simulink model "CF012A_GmStrtStop"  (R2013b)
settings: Solver=FixedStepDiscrete  SolverMode=SingleTasking  StartTime=0.0  StopTime=1  FixedStep=0.002  RelTol=1e-3
values from neighbouring files (symbols this model uses):
  CNV100MICROSECTOMILLISEC_MILLISECPERCNT_F32 = DataDict.Constant    [CF012A_GmStrtStop_DataDict.m]
  DISMOD_CNT_U08 = DataDict.Constant    [CF012A_GmStrtStop_DataDict.m]
  DISMODRATE_ULSPERSEC_F32 = DataDict.Constant    [CF012A_GmStrtStop_DataDict.m]
  FLTMOD_CNT_U08 = DataDict.Constant    [CF012A_GmStrtStop_DataDict.m]
  GmStrtStopEna = DataDict.Calibration    [CF012A_GmStrtStop_DataDict.m]
  GmStrtStopFltRateLim = DataDict.Calibration    [CF012A_GmStrtStop_DataDict.m]
  GmStrtStopMod1ToStopRateLim = DataDict.Calibration    [CF012A_GmStrtStop_DataDict.m]
  GmStrtStopNormRateLim = DataDict.Calibration    [CF012A_GmStrtStop_DataDict.m]
  GmStrtStopNormToMod1RateLim = DataDict.Calibration    [CF012A_GmStrtStop_DataDict.m]
  GmStrtStopStopAndMod2RateLim = DataDict.Calibration    [CF012A_GmStrtStop_DataDict.m]
  GmStrtStopStopMod1Tmr = DataDict.Calibration    [CF012A_GmStrtStop_DataDict.m]
  GmStrtStopStopMod2Tmr = DataDict.Calibration    [CF012A_GmStrtStop_DataDict.m]
  MOD1_CNT_U08 = DataDict.Constant    [CF012A_GmStrtStop_DataDict.m]
  MOD2_CNT_U08 = DataDict.Constant    [CF012A_GmStrtStop_DataDict.m]
  NORMMOD_CNT_U08 = DataDict.Constant    [CF012A_GmStrtStop_DataDict.m]
  STOPMOD_CNT_U08 = DataDict.Constant    [CF012A_GmStrtStop_DataDict.m]
  STRTSTOPRATEHILIM_ULSPERSEC_F32 = DataDict.Constant    [CF012A_GmStrtStop_DataDict.m]
  STRTSTOPRATELOWRLIM_ULSPERSEC_F32 = DataDict.Constant    [CF012A_GmStrtStop_DataDict.m]
  STRTSTOPSCAHILIM_ULS_F32 = DataDict.Constant    [CF012A_GmStrtStop_DataDict.m]
  STRTSTOPSCALOWRLIM_ULS_F32 = DataDict.Constant    [CF012A_GmStrtStop_DataDict.m]
undefined symbols (not defined in the file or in its folder): u2, u3, u4, u5
libraries: FixdToFloat x2, NxtrLim x2, simulink x2
(part 3 of 4)

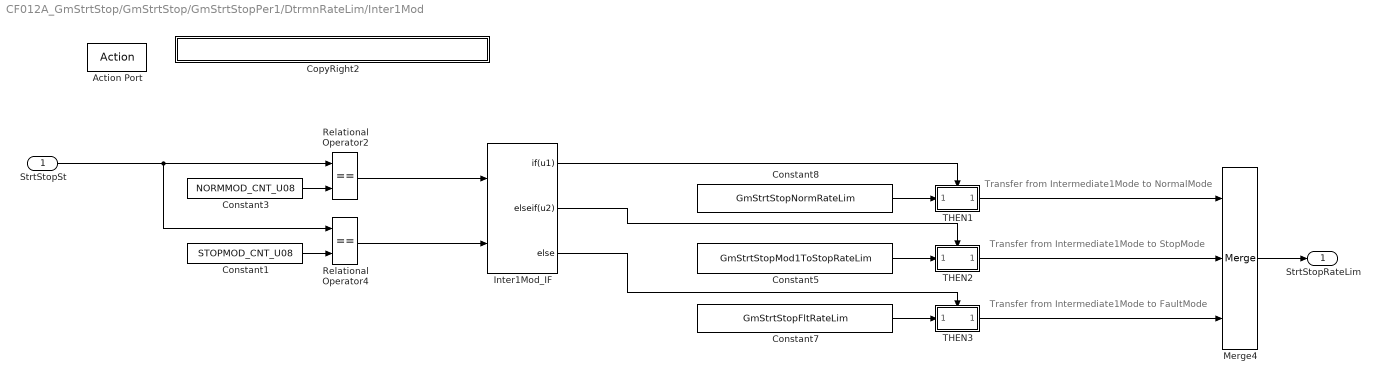
== system CF012A_GmStrtStop/GmStrtStop/GmStrtStopPer1/DtrmnRateLim/Inter1Mod ==
  note: Transfer from Intermediate1Mode to NormalMode
  note: Transfer from Intermediate1Mode to StopMode
  note: Transfer from Intermediate1Mode to FaultMode
  StrtStopSt : Inport  RequirementInfo="{'linktype_rmi_doors' '0000c6e0 (/GM T1XX/SubSystem Specifications/Customer Functions/CF012 12V Start Stop)' '#148' 'true' 'REQ:  148' '' } %GIDa_f5330e2e_2d56_43f6_8853_8fc29ce50161"
  Action Port : ActionPort  ActionType=elseif
  Constant1 : Constant  RequirementInfo="{'linktype_rmi_doors' '0000c6e0 (/GM T1XX/SubSystem Specifications/Customer Functions/CF012 12V Start Stop)' '#188' 'true' 'REQ:  188' '' } %GIDa_86f023b6_4738_45d0_828d_c113ed7026e9"  Value=STOPMOD_CNT_U08
  Constant3 : Constant  RequirementInfo="{'linktype_rmi_doors' '0000c6e0 (/GM T1XX/SubSystem Specifications/Customer Functions/CF012 12V Start Stop)' '#148' 'true' 'REQ:  148' '' } %GIDa_17212798_c997_48f1_a715_ee95a1adc504"  Value=NORMMOD_CNT_U08
  Constant5 : Constant  RequirementInfo="{'linktype_rmi_doors' '0000c6e0 (/GM T1XX/SubSystem Specifications/Customer Functions/CF012 12V Start Stop)' '#188' 'true' 'REQ:  188' '' } %GIDa_c9c10e63_8319_420b_bd57_9b2abca2294d"  Value=GmStrtStopMod1ToStopRateLim  OutDataTypeStr=single
  Constant7 : Constant  RequirementInfo="{'linktype_rmi_doors' '0000c6e0 (/GM T1XX/SubSystem Specifications/Customer Functions/CF012 12V Start Stop)' '#196' 'true' 'REQ:  196' '' } %GIDa_3c95a9bc_424d_44d0_af3d_886c4295a172"  Value=GmStrtStopFltRateLim  OutDataTypeStr=single
  Constant8 : Constant  RequirementInfo="{'linktype_rmi_doors' '0000c6e0 (/GM T1XX/SubSystem Specifications/Customer Functions/CF012 12V Start Stop)' '#148' 'true' 'REQ:  148' '' } %GIDa_b1015bd6_7f60_4122_9076_9e894186dcc2"  Value=GmStrtStopNormRateLim  OutDataTypeStr=single
  CopyRight2 : Subsystem  Description=|  mask(Copyright Information){none=on}
      | Copyright info block.                                               
      |                                                                     
      | Place copyright information at the top of every subsystem in design.
      mask prompts: none "No parameters"
      mask help: Place copyright information at the top of every subsystem in design.
      mask Display:
      | NxtrConf = 'Nexteer Confidential';
      | 
      | sys = bdroot; %handle for the current model ("system")
      | first = get_param(sys,'Created');
      | if(isempty(first))
      |     first = datestr(now,'yyyy');
      | else
      |     first = first(end-3:end);  %year is last four digits
      | end
      | 
      | last = get_param(sys,'LastModifiedDate');
      | if isempty(last)
      |     last = datestr(now,'yyyy');
      | else
      |     last = last(end-3:end);
      | end
      | 
      | if strcmp(first,last)
      |     fprintf('%s -- Copyright %s Nexteer',NxtrConf,first)
      | else
      |     fprintf('%s -- %s%s- %s Nexteer',NxtrConf,char(169),first,last)
      | end
  Inter1Mod_IF : If  RequirementInfo="{'linktype_rmi_doors' '0000c6e0 (/GM T1XX/SubSystem Specifications/Customer Functions/CF012 12V Start Stop)' '#148' 'true' 'REQ:  148' '' ; 'linktype_rmi_doors' '0000c6e0 (/GM T1XX/SubSystem Specifications/Customer Functions/CF012 12V Start Stop)' '#188' 'true' 'REQ:  188' '' ; 'linktype_rmi_doors' '0000c6e0 (/GM T1XX/SubSystem Specifications/Customer Functions/CF012 12V Start Stop)' '#196' 'true' 'REQ:  196' '' } %GIDa_bee18bf5_7cb1_484e_b310_4188a01c4900"  NumInputs=2  IfExpression=u1  ElseIfExpressions=u2
  Merge4 : Merge  RequirementInfo="{'linktype_rmi_doors' '0000c6e0 (/GM T1XX/SubSystem Specifications/Customer Functions/CF012 12V Start Stop)' '#148' 'true' 'REQ:  148' '' } %GIDa_b0435a17_739c_4c31_ac1a_85f448c6e576"  Inputs=3
  Relational Operator2 : RelationalOperator  RequirementInfo="{'linktype_rmi_doors' '0000c6e0 (/GM T1XX/SubSystem Specifications/Customer Functions/CF012 12V Start Stop)' '#148' 'true' 'REQ:  148' '' } %GIDa_db00afd9_8b52_48d0_ab8e_5bbb76a40030"  Operator===  OutDataTypeStr=boolean
  Relational Operator4 : RelationalOperator  RequirementInfo="{'linktype_rmi_doors' '0000c6e0 (/GM T1XX/SubSystem Specifications/Customer Functions/CF012 12V Start Stop)' '#188' 'true' 'REQ:  188' '' } %GIDa_101f5b8d_2727_47d9_95c5_fda015ecb9e6"  Operator===  OutDataTypeStr=boolean
  THEN1 : Subsystem  RequirementInfo="{'linktype_rmi_doors' '0000c6e0 (/GM T1XX/SubSystem Specifications/Customer Functions/CF012 12V Start Stop)' '#148' 'true' 'REQ:  148' '' } %GIDa_2f2a99d6_809f_487e_849d_5a2ecb99bded"  TreatAsAtomicUnit=on  mask(pass thru, version Nov 30, 2012){nIn=1}
      mask prompts: nIn "Number of input signals"
      mask help:
      | This block passes its input straight through without modification.
      |
      | Enter the number of signals to pass through (integer 1 to 5).
      mask Callback nIn:
      | thisBlock = gcb;
      | a = get_param(thisBlock,'MaskValues');
      | b = cell2mat(a);
      | c = str2num(b);
      | 
      | if c<1 c=1; end
      | if c>5 c=5; end
      | 
      | for idx=1:c
      |     sIdx = num2str(idx);
      |     oldblock = [thisBlock '/In' sIdx];
      |     if strcmp(get_param(oldblock,'BlockType'),'Ground')
      |          newblock = 'built-in/Inport';
      |         pos = get_param(oldblock,'Position');
      |         orient = get_param(oldblock,'Orientation');
      |         delete_block(oldblock);
      |         add_block(newblock,oldblock,'Position',pos, 'Orientation',orient);
      |     end
      | 
      |     oldblock = [thisBlock '/Out' sIdx];
      |     if strcmp(get_param(oldblock,'BlockType'),'Terminator')
      |         newblock = 'built-in/Outport';
      |         pos = get_param(oldblock,'Position');
      |         orient = get_param(oldblock,'Orientation');
      |         delete_block(oldblock);
      |         add_block(newblock,oldblock,'Position',pos, 'Orientation',orient);
      |     end
      | end
      | 
      | for idx=c+1:5
      |     sIdx = num2str(idx);
      |     oldblock = [thisBlock '/In' sIdx];
      |     if strcmp(get_param(oldblock,'BlockType'),'Inport')
      |         newblock = 'built-in/Ground';
      |         pos = get_param(oldblock,'Position');
      |         orient = get_param(oldblock,'Orientation');
      |         delete_block(oldblock);
      |         add_block(newblock,oldblock,'Position',pos, 'Orientation',orient);
      |     end
      | 
      |     oldblock = [thisBlock '/Out' sIdx];
      |     if strcmp(get_param(oldblock,'BlockType'),'Outport')
      |         newblock = 'built-in/Terminator';
      |         pos = get_param(oldblock,'Position');
      |         orient = get_param(oldblock,'Orientation');
      |         delete_block(oldblock);
      |         add_block(newblock,oldblock,'Position',pos, 'Orientation',orient);
      |     end
      | end
      | 
      | 
      | 
      | clear thisBlock oldblock newblock orient pos a b c idx sIdx ;
      mask Display: fprintf('pass\nthru')
  THEN2 : Subsystem  RequirementInfo="{'linktype_rmi_doors' '0000c6e0 (/GM T1XX/SubSystem Specifications/Customer Functions/CF012 12V Start Stop)' '#188' 'true' 'REQ:  188' '' } %GIDa_b2d571eb_81f6_48b0_94ac_681d473bd688"  TreatAsAtomicUnit=on  mask(pass thru, version Nov 30, 2012){nIn=1}
      mask prompts: nIn "Number of input signals"
      mask help:
      | This block passes its input straight through without modification.
      |
      | Enter the number of signals to pass through (integer 1 to 5).
      mask Callback nIn:
      | thisBlock = gcb;
      | a = get_param(thisBlock,'MaskValues');
      | b = cell2mat(a);
      | c = str2num(b);
      | 
      | if c<1 c=1; end
      | if c>5 c=5; end
      | 
      | for idx=1:c
      |     sIdx = num2str(idx);
      |     oldblock = [thisBlock '/In' sIdx];
      |     if strcmp(get_param(oldblock,'BlockType'),'Ground')
      |          newblock = 'built-in/Inport';
      |         pos = get_param(oldblock,'Position');
      |         orient = get_param(oldblock,'Orientation');
      |         delete_block(oldblock);
      |         add_block(newblock,oldblock,'Position',pos, 'Orientation',orient);
      |     end
      | 
      |     oldblock = [thisBlock '/Out' sIdx];
      |     if strcmp(get_param(oldblock,'BlockType'),'Terminator')
      |         newblock = 'built-in/Outport';
      |         pos = get_param(oldblock,'Position');
      |         orient = get_param(oldblock,'Orientation');
      |         delete_block(oldblock);
      |         add_block(newblock,oldblock,'Position',pos, 'Orientation',orient);
      |     end
      | end
      | 
      | for idx=c+1:5
      |     sIdx = num2str(idx);
      |     oldblock = [thisBlock '/In' sIdx];
      |     if strcmp(get_param(oldblock,'BlockType'),'Inport')
      |         newblock = 'built-in/Ground';
      |         pos = get_param(oldblock,'Position');
      |         orient = get_param(oldblock,'Orientation');
      |         delete_block(oldblock);
      |         add_block(newblock,oldblock,'Position',pos, 'Orientation',orient);
      |     end
      | 
      |     oldblock = [thisBlock '/Out' sIdx];
      |     if strcmp(get_param(oldblock,'BlockType'),'Outport')
      |         newblock = 'built-in/Terminator';
      |         pos = get_param(oldblock,'Position');
      |         orient = get_param(oldblock,'Orientation');
      |         delete_block(oldblock);
      |         add_block(newblock,oldblock,'Position',pos, 'Orientation',orient);
      |     end
      | end
      | 
      | 
      | 
      | clear thisBlock oldblock newblock orient pos a b c idx sIdx ;
      mask Display: fprintf('pass\nthru')
  THEN3 : Subsystem  RequirementInfo="{'linktype_rmi_doors' '0000c6e0 (/GM T1XX/SubSystem Specifications/Customer Functions/CF012 12V Start Stop)' '#196' 'true' 'REQ:  196' '' } %GIDa_eb12a114_e698_478c_8ca5_615ae26c6696"  TreatAsAtomicUnit=on  mask(pass thru, version Nov 30, 2012){nIn=1}
      mask prompts: nIn "Number of input signals"
      mask help:
      | This block passes its input straight through without modification.
      |
      | Enter the number of signals to pass through (integer 1 to 5).
      mask Callback nIn:
      | thisBlock = gcb;
      | a = get_param(thisBlock,'MaskValues');
      | b = cell2mat(a);
      | c = str2num(b);
      | 
      | if c<1 c=1; end
      | if c>5 c=5; end
      | 
      | for idx=1:c
      |     sIdx = num2str(idx);
      |     oldblock = [thisBlock '/In' sIdx];
      |     if strcmp(get_param(oldblock,'BlockType'),'Ground')
      |          newblock = 'built-in/Inport';
      |         pos = get_param(oldblock,'Position');
      |         orient = get_param(oldblock,'Orientation');
      |         delete_block(oldblock);
      |         add_block(newblock,oldblock,'Position',pos, 'Orientation',orient);
      |     end
      | 
      |     oldblock = [thisBlock '/Out' sIdx];
      |     if strcmp(get_param(oldblock,'BlockType'),'Terminator')
      |         newblock = 'built-in/Outport';
      |         pos = get_param(oldblock,'Position');
      |         orient = get_param(oldblock,'Orientation');
      |         delete_block(oldblock);
      |         add_block(newblock,oldblock,'Position',pos, 'Orientation',orient);
      |     end
      | end
      | 
      | for idx=c+1:5
      |     sIdx = num2str(idx);
      |     oldblock = [thisBlock '/In' sIdx];
      |     if strcmp(get_param(oldblock,'BlockType'),'Inport')
      |         newblock = 'built-in/Ground';
      |         pos = get_param(oldblock,'Position');
      |         orient = get_param(oldblock,'Orientation');
      |         delete_block(oldblock);
      |         add_block(newblock,oldblock,'Position',pos, 'Orientation',orient);
      |     end
      | 
      |     oldblock = [thisBlock '/Out' sIdx];
      |     if strcmp(get_param(oldblock,'BlockType'),'Outport')
      |         newblock = 'built-in/Terminator';
      |         pos = get_param(oldblock,'Position');
      |         orient = get_param(oldblock,'Orientation');
      |         delete_block(oldblock);
      |         add_block(newblock,oldblock,'Position',pos, 'Orientation',orient);
      |     end
      | end
      | 
      | 
      | 
      | clear thisBlock oldblock newblock orient pos a b c idx sIdx ;
      mask Display: fprintf('pass\nthru')
  StrtStopRateLim : Outport  RequirementInfo="{'linktype_rmi_doors' '0000c6e0 (/GM T1XX/SubSystem Specifications/Customer Functions/CF012 12V Start Stop)' '#148' 'true' 'REQ:  148' '' } %GIDa_327ececa_8699_4446_8fde_5bf9f2022ae5"
  wires:
  Merge4/1 -> StrtStopRateLim/1
  Constant8/1 -> THEN1/1(In1)
  Constant5/1 -> THEN2/1(In1)
  Constant7/1 -> THEN3/1(In1)
  StrtStopSt/1 -> Relational Operator4/1, Relational Operator2/1
  Inter1Mod_IF/2 -> THEN2/Action
  THEN1/1(Out1) -> Merge4/1
  THEN2/1(Out1) -> Merge4/2
  Inter1Mod_IF/1 -> THEN1/Action
  THEN3/1(Out1) -> Merge4/3
  Inter1Mod_IF/3 -> THEN3/Action
  Constant3/1 -> Relational Operator2/2
  Constant1/1 -> Relational Operator4/2
  Relational Operator2/1 -> Inter1Mod_IF/1
  Relational Operator4/1 -> Inter1Mod_IF/2

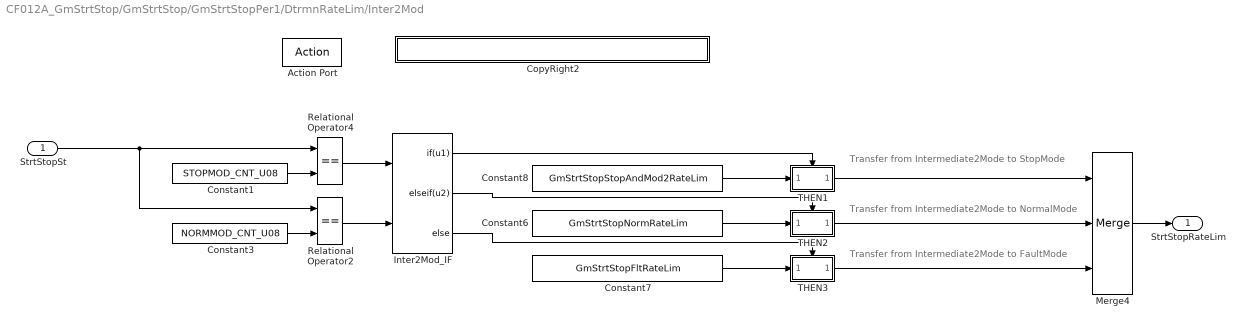
== system CF012A_GmStrtStop/GmStrtStop/GmStrtStopPer1/DtrmnRateLim/Inter2Mod ==
  note: Transfer from Intermediate2Mode to StopMode
  note: Transfer from Intermediate2Mode to NormalMode
  note: Transfer from Intermediate2Mode to FaultMode
  StrtStopSt : Inport
  Action Port : ActionPort  ActionType=elseif
  Constant1 : Constant  RequirementInfo="{'linktype_rmi_doors' '0000c6e0 (/GM T1XX/SubSystem Specifications/Customer Functions/CF012 12V Start Stop)' '#191' 'true' 'REQ:  191' '' } %GIDa_a83bcf33_e1ed_436f_96b3_5797f72692a7"  Value=STOPMOD_CNT_U08
  Constant3 : Constant  RequirementInfo="{'linktype_rmi_doors' '0000c6e0 (/GM T1XX/SubSystem Specifications/Customer Functions/CF012 12V Start Stop)' '#165' 'true' 'REQ:  165' '' } %GIDa_8085c648_06a7_45a7_9255_7980080a1e3b"  Value=NORMMOD_CNT_U08
  Constant6 : Constant  RequirementInfo="{'linktype_rmi_doors' '0000c6e0 (/GM T1XX/SubSystem Specifications/Customer Functions/CF012 12V Start Stop)' '#165' 'true' 'REQ:  165' '' } %GIDa_9243c5b2_93a6_4816_a712_340b316f07e9"  Value=GmStrtStopNormRateLim  OutDataTypeStr=single
  Constant7 : Constant  RequirementInfo="{'linktype_rmi_doors' '0000c6e0 (/GM T1XX/SubSystem Specifications/Customer Functions/CF012 12V Start Stop)' '#196' 'true' 'REQ:  196' '' } %GIDa_8581bb06_cdfa_4b6e_b4f2_29ada5e81c3a"  Value=GmStrtStopFltRateLim  OutDataTypeStr=single
  Constant8 : Constant  RequirementInfo="{'linktype_rmi_doors' '0000c6e0 (/GM T1XX/SubSystem Specifications/Customer Functions/CF012 12V Start Stop)' '#191' 'true' 'REQ:  191' '' } %GIDa_3cce6931_1fb4_4063_9bce_15191e06056a"  Value=GmStrtStopStopAndMod2RateLim  OutDataTypeStr=single
  CopyRight2 : Subsystem  Description=|  mask(Copyright Information){none=on}
      | Copyright info block.                                               
      |                                                                     
      | Place copyright information at the top of every subsystem in design.
      mask prompts: none "No parameters"
      mask help: Place copyright information at the top of every subsystem in design.
      mask Display:
      | NxtrConf = 'Nexteer Confidential';
      | 
      | sys = bdroot; %handle for the current model ("system")
      | first = get_param(sys,'Created');
      | if(isempty(first))
      |     first = datestr(now,'yyyy');
      | else
      |     first = first(end-3:end);  %year is last four digits
      | end
      | 
      | last = get_param(sys,'LastModifiedDate');
      | if isempty(last)
      |     last = datestr(now,'yyyy');
      | else
      |     last = last(end-3:end);
      | end
      | 
      | if strcmp(first,last)
      |     fprintf('%s -- Copyright %s Nexteer',NxtrConf,first)
      | else
      |     fprintf('%s -- %s%s- %s Nexteer',NxtrConf,char(169),first,last)
      | end
  Inter2Mod_IF : If  RequirementInfo="{'linktype_rmi_doors' '0000c6e0 (/GM T1XX/SubSystem Specifications/Customer Functions/CF012 12V Start Stop)' '#165' 'true' 'REQ:  165' '' ; 'linktype_rmi_doors' '0000c6e0 (/GM T1XX/SubSystem Specifications/Customer Functions/CF012 12V Start Stop)' '#196' 'true' 'REQ:  196' '' ; 'linktype_rmi_doors' '0000c6e0 (/GM T1XX/SubSystem Specifications/Customer Functions/CF012 12V Start Stop)' '#191' 'true' 'REQ:  191' '' } %GIDa_6bb53297_5842_4dfb_a8ef_f350d77e5822"  NumInputs=2  IfExpression=u1  ElseIfExpressions=u2
  Merge4 : Merge  Inputs=3
  Relational Operator2 : RelationalOperator  RequirementInfo="{'linktype_rmi_doors' '0000c6e0 (/GM T1XX/SubSystem Specifications/Customer Functions/CF012 12V Start Stop)' '#165' 'true' 'REQ:  165' '' } %GIDa_08db98e9_f714_4dca_ae7e_f32727df577e"  Operator===  OutDataTypeStr=boolean
  Relational Operator4 : RelationalOperator  RequirementInfo="{'linktype_rmi_doors' '0000c6e0 (/GM T1XX/SubSystem Specifications/Customer Functions/CF012 12V Start Stop)' '#191' 'true' 'REQ:  191' '' } %GIDa_01fbe4bd_96c5_4845_9d8c_3914e66803a3"  Operator===  OutDataTypeStr=boolean
  THEN1 : Subsystem  RequirementInfo="{'linktype_rmi_doors' '0000c6e0 (/GM T1XX/SubSystem Specifications/Customer Functions/CF012 12V Start Stop)' '#191' 'true' 'REQ:  191' '' } %GIDa_125c63d8_a60e_4bd1_9a24_ee09e1ad26f8"  TreatAsAtomicUnit=on  mask(pass thru, version Nov 30, 2012){nIn=1}
      mask prompts: nIn "Number of input signals"
      mask help:
      | This block passes its input straight through without modification.
      |
      | Enter the number of signals to pass through (integer 1 to 5).
      mask Callback nIn:
      | thisBlock = gcb;
      | a = get_param(thisBlock,'MaskValues');
      | b = cell2mat(a);
      | c = str2num(b);
      | 
      | if c<1 c=1; end
      | if c>5 c=5; end
      | 
      | for idx=1:c
      |     sIdx = num2str(idx);
      |     oldblock = [thisBlock '/In' sIdx];
      |     if strcmp(get_param(oldblock,'BlockType'),'Ground')
      |          newblock = 'built-in/Inport';
      |         pos = get_param(oldblock,'Position');
      |         orient = get_param(oldblock,'Orientation');
      |         delete_block(oldblock);
      |         add_block(newblock,oldblock,'Position',pos, 'Orientation',orient);
      |     end
      | 
      |     oldblock = [thisBlock '/Out' sIdx];
      |     if strcmp(get_param(oldblock,'BlockType'),'Terminator')
      |         newblock = 'built-in/Outport';
      |         pos = get_param(oldblock,'Position');
      |         orient = get_param(oldblock,'Orientation');
      |         delete_block(oldblock);
      |         add_block(newblock,oldblock,'Position',pos, 'Orientation',orient);
      |     end
      | end
      | 
      | for idx=c+1:5
      |     sIdx = num2str(idx);
      |     oldblock = [thisBlock '/In' sIdx];
      |     if strcmp(get_param(oldblock,'BlockType'),'Inport')
      |         newblock = 'built-in/Ground';
      |         pos = get_param(oldblock,'Position');
      |         orient = get_param(oldblock,'Orientation');
      |         delete_block(oldblock);
      |         add_block(newblock,oldblock,'Position',pos, 'Orientation',orient);
      |     end
      | 
      |     oldblock = [thisBlock '/Out' sIdx];
      |     if strcmp(get_param(oldblock,'BlockType'),'Outport')
      |         newblock = 'built-in/Terminator';
      |         pos = get_param(oldblock,'Position');
      |         orient = get_param(oldblock,'Orientation');
      |         delete_block(oldblock);
      |         add_block(newblock,oldblock,'Position',pos, 'Orientation',orient);
      |     end
      | end
      | 
      | 
      | 
      | clear thisBlock oldblock newblock orient pos a b c idx sIdx ;
      mask Display: fprintf('pass\nthru')
  THEN2 : Subsystem  RequirementInfo="{'linktype_rmi_doors' '0000c6e0 (/GM T1XX/SubSystem Specifications/Customer Functions/CF012 12V Start Stop)' '#165' 'true' 'REQ:  165' '' } %GIDa_d431bc61_ac2d_4eb9_b60b_66a4661bbd0d"  TreatAsAtomicUnit=on  mask(pass thru, version Nov 30, 2012){nIn=1}
      mask prompts: nIn "Number of input signals"
      mask help:
      | This block passes its input straight through without modification.
      |
      | Enter the number of signals to pass through (integer 1 to 5).
      mask Callback nIn:
      | thisBlock = gcb;
      | a = get_param(thisBlock,'MaskValues');
      | b = cell2mat(a);
      | c = str2num(b);
      | 
      | if c<1 c=1; end
      | if c>5 c=5; end
      | 
      | for idx=1:c
      |     sIdx = num2str(idx);
      |     oldblock = [thisBlock '/In' sIdx];
      |     if strcmp(get_param(oldblock,'BlockType'),'Ground')
      |          newblock = 'built-in/Inport';
      |         pos = get_param(oldblock,'Position');
      |         orient = get_param(oldblock,'Orientation');
      |         delete_block(oldblock);
      |         add_block(newblock,oldblock,'Position',pos, 'Orientation',orient);
      |     end
      | 
      |     oldblock = [thisBlock '/Out' sIdx];
      |     if strcmp(get_param(oldblock,'BlockType'),'Terminator')
      |         newblock = 'built-in/Outport';
      |         pos = get_param(oldblock,'Position');
      |         orient = get_param(oldblock,'Orientation');
      |         delete_block(oldblock);
      |         add_block(newblock,oldblock,'Position',pos, 'Orientation',orient);
      |     end
      | end
      | 
      | for idx=c+1:5
      |     sIdx = num2str(idx);
      |     oldblock = [thisBlock '/In' sIdx];
      |     if strcmp(get_param(oldblock,'BlockType'),'Inport')
      |         newblock = 'built-in/Ground';
      |         pos = get_param(oldblock,'Position');
      |         orient = get_param(oldblock,'Orientation');
      |         delete_block(oldblock);
      |         add_block(newblock,oldblock,'Position',pos, 'Orientation',orient);
      |     end
      | 
      |     oldblock = [thisBlock '/Out' sIdx];
      |     if strcmp(get_param(oldblock,'BlockType'),'Outport')
      |         newblock = 'built-in/Terminator';
      |         pos = get_param(oldblock,'Position');
      |         orient = get_param(oldblock,'Orientation');
      |         delete_block(oldblock);
      |         add_block(newblock,oldblock,'Position',pos, 'Orientation',orient);
      |     end
      | end
      | 
      | 
      | 
      | clear thisBlock oldblock newblock orient pos a b c idx sIdx ;
      mask Display: fprintf('pass\nthru')
  THEN3 : Subsystem  RequirementInfo="{'linktype_rmi_doors' '0000c6e0 (/GM T1XX/SubSystem Specifications/Customer Functions/CF012 12V Start Stop)' '#196' 'true' 'REQ:  196' '' } %GIDa_d274ed7f_1790_4473_a30d_b91f86cccf9c"  TreatAsAtomicUnit=on  mask(pass thru, version Nov 30, 2012){nIn=1}
      mask prompts: nIn "Number of input signals"
      mask help:
      | This block passes its input straight through without modification.
      |
      | Enter the number of signals to pass through (integer 1 to 5).
      mask Callback nIn:
      | thisBlock = gcb;
      | a = get_param(thisBlock,'MaskValues');
      | b = cell2mat(a);
      | c = str2num(b);
      | 
      | if c<1 c=1; end
      | if c>5 c=5; end
      | 
      | for idx=1:c
      |     sIdx = num2str(idx);
      |     oldblock = [thisBlock '/In' sIdx];
      |     if strcmp(get_param(oldblock,'BlockType'),'Ground')
      |          newblock = 'built-in/Inport';
      |         pos = get_param(oldblock,'Position');
      |         orient = get_param(oldblock,'Orientation');
      |         delete_block(oldblock);
      |         add_block(newblock,oldblock,'Position',pos, 'Orientation',orient);
      |     end
      | 
      |     oldblock = [thisBlock '/Out' sIdx];
      |     if strcmp(get_param(oldblock,'BlockType'),'Terminator')
      |         newblock = 'built-in/Outport';
      |         pos = get_param(oldblock,'Position');
      |         orient = get_param(oldblock,'Orientation');
      |         delete_block(oldblock);
      |         add_block(newblock,oldblock,'Position',pos, 'Orientation',orient);
      |     end
      | end
      | 
      | for idx=c+1:5
      |     sIdx = num2str(idx);
      |     oldblock = [thisBlock '/In' sIdx];
      |     if strcmp(get_param(oldblock,'BlockType'),'Inport')
      |         newblock = 'built-in/Ground';
      |         pos = get_param(oldblock,'Position');
      |         orient = get_param(oldblock,'Orientation');
      |         delete_block(oldblock);
      |         add_block(newblock,oldblock,'Position',pos, 'Orientation',orient);
      |     end
      | 
      |     oldblock = [thisBlock '/Out' sIdx];
      |     if strcmp(get_param(oldblock,'BlockType'),'Outport')
      |         newblock = 'built-in/Terminator';
      |         pos = get_param(oldblock,'Position');
      |         orient = get_param(oldblock,'Orientation');
      |         delete_block(oldblock);
      |         add_block(newblock,oldblock,'Position',pos, 'Orientation',orient);
      |     end
      | end
      | 
      | 
      | 
      | clear thisBlock oldblock newblock orient pos a b c idx sIdx ;
      mask Display: fprintf('pass\nthru')
  StrtStopRateLim : Outport
  wires:
  Constant7/1 -> THEN3/1(In1)
  Constant6/1 -> THEN2/1(In1)
  Constant8/1 -> THEN1/1(In1)
  Merge4/1 -> StrtStopRateLim/1
  Inter2Mod_IF/2 -> THEN2/Action
  THEN1/1(Out1) -> Merge4/1
  THEN2/1(Out1) -> Merge4/2
  Inter2Mod_IF/1 -> THEN1/Action
  THEN3/1(Out1) -> Merge4/3
  Inter2Mod_IF/3 -> THEN3/Action
  StrtStopSt/1 -> Relational Operator2/1, Relational Operator4/1
  Constant3/1 -> Relational Operator2/2
  Constant1/1 -> Relational Operator4/2
  Relational Operator4/1 -> Inter2Mod_IF/1
  Relational Operator2/1 -> Inter2Mod_IF/2

== system CF012A_GmStrtStop/GmStrtStop/GmStrtStopPer1/DtrmnRateLim/NormMod ==
  note: Transfer from NormalMode to Intermediate1Mode
  note: Transfer from NormalMode to FaultMode
  StrtStopSt : Inport
  Action Port : ActionPort  ActionType=then
  Constant1 : Constant  RequirementInfo="{'linktype_rmi_doors' '0000c6e0 (/GM T1XX/SubSystem Specifications/Customer Functions/CF012 12V Start Stop)' '#186' 'true' 'REQ:  186' '' } %GIDa_dfcbd125_64a6_4974_8244_63706063c233"  Value=MOD1_CNT_U08
  Constant4 : Constant  RequirementInfo="{'linktype_rmi_doors' '0000c6e0 (/GM T1XX/SubSystem Specifications/Customer Functions/CF012 12V Start Stop)' '#196' 'true' 'REQ:  196' '' } %GIDa_eab5f001_d033_4082_9bae_0911224d14c1"  Value=GmStrtStopFltRateLim  OutDataTypeStr=single
  Constant8 : Constant  RequirementInfo="{'linktype_rmi_doors' '0000c6e0 (/GM T1XX/SubSystem Specifications/Customer Functions/CF012 12V Start Stop)' '#186' 'true' 'REQ:  186' '' } %GIDa_bdd6fe5a_920d_465a_ab34_47b9f0995da1"  Value=GmStrtStopNormToMod1RateLim  OutDataTypeStr=single
  CopyRight2 : Subsystem  Description=|  mask(Copyright Information){none=on}
      | Copyright info block.                                               
      |                                                                     
      | Place copyright information at the top of every subsystem in design.
      mask prompts: none "No parameters"
      mask help: Place copyright information at the top of every subsystem in design.
      mask Display:
      | NxtrConf = 'Nexteer Confidential';
      | 
      | sys = bdroot; %handle for the current model ("system")
      | first = get_param(sys,'Created');
      | if(isempty(first))
      |     first = datestr(now,'yyyy');
      | else
      |     first = first(end-3:end);  %year is last four digits
      | end
      | 
      | last = get_param(sys,'LastModifiedDate');
      | if isempty(last)
      |     last = datestr(now,'yyyy');
      | else
      |     last = last(end-3:end);
      | end
      | 
      | if strcmp(first,last)
      |     fprintf('%s -- Copyright %s Nexteer',NxtrConf,first)
      | else
      |     fprintf('%s -- %s%s- %s Nexteer',NxtrConf,char(169),first,last)
      | end
  Merge1 : Merge  RequirementInfo="{'linktype_rmi_doors' '0000c6e0 (/GM T1XX/SubSystem Specifications/Customer Functions/CF012 12V Start Stop)' '#186' 'true' 'REQ:  186' '' } %GIDa_96cdee7c_d581_420d_be25_2a15d1578a0e"
  NormMod_IF : If  RequirementInfo="{'linktype_rmi_doors' '0000c6e0 (/GM T1XX/SubSystem Specifications/Customer Functions/CF012 12V Start Stop)' '#186' 'true' 'REQ:  186' '' ; 'linktype_rmi_doors' '0000c6e0 (/GM T1XX/SubSystem Specifications/Customer Functions/CF012 12V Start Stop)' '#196' 'true' 'REQ:  196' '' } %GIDa_9c436332_0426_4999_a176_97e2475f85f1"  IfExpression=u1
  Relational Operator3 : RelationalOperator  RequirementInfo="{'linktype_rmi_doors' '0000c6e0 (/GM T1XX/SubSystem Specifications/Customer Functions/CF012 12V Start Stop)' '#186' 'true' 'REQ:  186' '' } %GIDa_bc842b73_e87d_428b_b363_05cdd27f8702"  Operator===  OutDataTypeStr=boolean
  THEN3 : Subsystem  RequirementInfo="{'linktype_rmi_doors' '0000c6e0 (/GM T1XX/SubSystem Specifications/Customer Functions/CF012 12V Start Stop)' '#186' 'true' 'REQ:  186' '' } %GIDa_c59beb66_0cc7_44d7_a17d_7635f6f08bb4"  TreatAsAtomicUnit=on  mask(pass thru, version Nov 30, 2012){nIn=1}
      mask prompts: nIn "Number of input signals"
      mask help:
      | This block passes its input straight through without modification.
      |
      | Enter the number of signals to pass through (integer 1 to 5).
      mask Callback nIn:
      | thisBlock = gcb;
      | a = get_param(thisBlock,'MaskValues');
      | b = cell2mat(a);
      | c = str2num(b);
      | 
      | if c<1 c=1; end
      | if c>5 c=5; end
      | 
      | for idx=1:c
      |     sIdx = num2str(idx);
      |     oldblock = [thisBlock '/In' sIdx];
      |     if strcmp(get_param(oldblock,'BlockType'),'Ground')
      |          newblock = 'built-in/Inport';
      |         pos = get_param(oldblock,'Position');
      |         orient = get_param(oldblock,'Orientation');
      |         delete_block(oldblock);
      |         add_block(newblock,oldblock,'Position',pos, 'Orientation',orient);
      |     end
      | 
      |     oldblock = [thisBlock '/Out' sIdx];
      |     if strcmp(get_param(oldblock,'BlockType'),'Terminator')
      |         newblock = 'built-in/Outport';
      |         pos = get_param(oldblock,'Position');
      |         orient = get_param(oldblock,'Orientation');
      |         delete_block(oldblock);
      |         add_block(newblock,oldblock,'Position',pos, 'Orientation',orient);
      |     end
      | end
      | 
      | for idx=c+1:5
      |     sIdx = num2str(idx);
      |     oldblock = [thisBlock '/In' sIdx];
      |     if strcmp(get_param(oldblock,'BlockType'),'Inport')
      |         newblock = 'built-in/Ground';
      |         pos = get_param(oldblock,'Position');
      |         orient = get_param(oldblock,'Orientation');
      |         delete_block(oldblock);
      |         add_block(newblock,oldblock,'Position',pos, 'Orientation',orient);
      |     end
      | 
      |     oldblock = [thisBlock '/Out' sIdx];
      |     if strcmp(get_param(oldblock,'BlockType'),'Outport')
      |         newblock = 'built-in/Terminator';
      |         pos = get_param(oldblock,'Position');
      |         orient = get_param(oldblock,'Orientation');
      |         delete_block(oldblock);
      |         add_block(newblock,oldblock,'Position',pos, 'Orientation',orient);
      |     end
      | end
      | 
      | 
      | 
      | clear thisBlock oldblock newblock orient pos a b c idx sIdx ;
      mask Display: fprintf('pass\nthru')
  THEN4 : Subsystem  RequirementInfo="{'linktype_rmi_doors' '0000c6e0 (/GM T1XX/SubSystem Specifications/Customer Functions/CF012 12V Start Stop)' '#196' 'true' 'REQ:  196' '' } %GIDa_2d08ff30_20b9_4675_9acb_0f33e4eb80cd"  TreatAsAtomicUnit=on  mask(pass thru, version Nov 30, 2012){nIn=1}
      mask prompts: nIn "Number of input signals"
      mask help:
      | This block passes its input straight through without modification.
      |
      | Enter the number of signals to pass through (integer 1 to 5).
      mask Callback nIn:
      | thisBlock = gcb;
      | a = get_param(thisBlock,'MaskValues');
      | b = cell2mat(a);
      | c = str2num(b);
      | 
      | if c<1 c=1; end
      | if c>5 c=5; end
      | 
      | for idx=1:c
      |     sIdx = num2str(idx);
      |     oldblock = [thisBlock '/In' sIdx];
      |     if strcmp(get_param(oldblock,'BlockType'),'Ground')
      |          newblock = 'built-in/Inport';
      |         pos = get_param(oldblock,'Position');
      |         orient = get_param(oldblock,'Orientation');
      |         delete_block(oldblock);
      |         add_block(newblock,oldblock,'Position',pos, 'Orientation',orient);
      |     end
      | 
      |     oldblock = [thisBlock '/Out' sIdx];
      |     if strcmp(get_param(oldblock,'BlockType'),'Terminator')
      |         newblock = 'built-in/Outport';
      |         pos = get_param(oldblock,'Position');
      |         orient = get_param(oldblock,'Orientation');
      |         delete_block(oldblock);
      |         add_block(newblock,oldblock,'Position',pos, 'Orientation',orient);
      |     end
      | end
      | 
      | for idx=c+1:5
      |     sIdx = num2str(idx);
      |     oldblock = [thisBlock '/In' sIdx];
      |     if strcmp(get_param(oldblock,'BlockType'),'Inport')
      |         newblock = 'built-in/Ground';
      |         pos = get_param(oldblock,'Position');
      |         orient = get_param(oldblock,'Orientation');
      |         delete_block(oldblock);
      |         add_block(newblock,oldblock,'Position',pos, 'Orientation',orient);
      |     end
      | 
      |     oldblock = [thisBlock '/Out' sIdx];
      |     if strcmp(get_param(oldblock,'BlockType'),'Outport')
      |         newblock = 'built-in/Terminator';
      |         pos = get_param(oldblock,'Position');
      |         orient = get_param(oldblock,'Orientation');
      |         delete_block(oldblock);
      |         add_block(newblock,oldblock,'Position',pos, 'Orientation',orient);
      |     end
      | end
      | 
      | 
      | 
      | clear thisBlock oldblock newblock orient pos a b c idx sIdx ;
      mask Display: fprintf('pass\nthru')
  StrtStopRateLim : Outport
  wires:
  Merge1/1 -> StrtStopRateLim/1
  NormMod_IF/2 -> THEN4/Action
  Constant4/1 -> THEN4/1(In1)
  Constant8/1 -> THEN3/1(In1)
  THEN3/1(Out1) -> Merge1/1
  THEN4/1(Out1) -> Merge1/2
  NormMod_IF/1 -> THEN3/Action
  Relational Operator3/1 -> NormMod_IF/1
  StrtStopSt/1 -> Relational Operator3/1
  Constant1/1 -> Relational Operator3/2

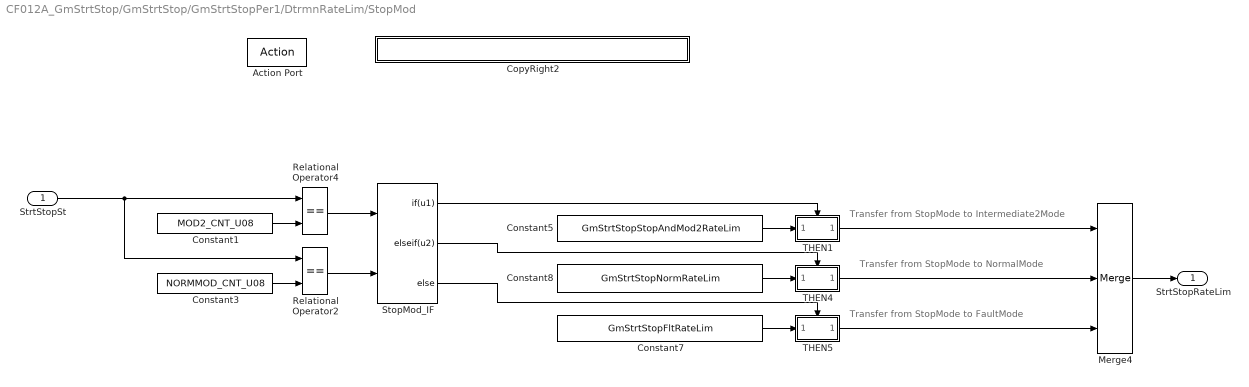
== system CF012A_GmStrtStop/GmStrtStop/GmStrtStopPer1/DtrmnRateLim/StopMod ==
  note: Transfer from StopMode to Intermediate2Mode
  note: Transfer from StopMode to NormalMode
  note: Transfer from StopMode to FaultMode
  StrtStopSt : Inport
  Action Port : ActionPort  ActionType=elseif
  Constant1 : Constant  RequirementInfo="{'linktype_rmi_doors' '0000c6e0 (/GM T1XX/SubSystem Specifications/Customer Functions/CF012 12V Start Stop)' '#191' 'true' 'REQ:  191' '' } %GIDa_f349c4b9_5951_45d5_aeee_6f74b3f6af33"  Value=MOD2_CNT_U08
  Constant3 : Constant  RequirementInfo="{'linktype_rmi_doors' '0000c6e0 (/GM T1XX/SubSystem Specifications/Customer Functions/CF012 12V Start Stop)' '#190' 'true' 'REQ:  190' '' } %GIDa_34eb844a_d2be_4f74_98ee_dacf5d19992e"  Value=NORMMOD_CNT_U08
  Constant5 : Constant  RequirementInfo="{'linktype_rmi_doors' '0000c6e0 (/GM T1XX/SubSystem Specifications/Customer Functions/CF012 12V Start Stop)' '#191' 'true' 'REQ:  191' '' } %GIDa_f2db297a_0015_417d_a43e_48699d2c3486"  Value=GmStrtStopStopAndMod2RateLim  OutDataTypeStr=single
  Constant7 : Constant  RequirementInfo="{'linktype_rmi_doors' '0000c6e0 (/GM T1XX/SubSystem Specifications/Customer Functions/CF012 12V Start Stop)' '#196' 'true' 'REQ:  196' '' } %GIDa_c6b4af8d_f267_4cc8_9f82_4d9a9f99c803"  Value=GmStrtStopFltRateLim  OutDataTypeStr=single
  Constant8 : Constant  RequirementInfo="{'linktype_rmi_doors' '0000c6e0 (/GM T1XX/SubSystem Specifications/Customer Functions/CF012 12V Start Stop)' '#190' 'true' 'REQ:  190' '' } %GIDa_03ab565a_dcf3_4915_85ef_cbc5ad876218"  Value=GmStrtStopNormRateLim  OutDataTypeStr=single
  CopyRight2 : Subsystem  Description=|  mask(Copyright Information){none=on}
      | Copyright info block.                                               
      |                                                                     
      | Place copyright information at the top of every subsystem in design.
      mask prompts: none "No parameters"
      mask help: Place copyright information at the top of every subsystem in design.
      mask Display:
      | NxtrConf = 'Nexteer Confidential';
      | 
      | sys = bdroot; %handle for the current model ("system")
      | first = get_param(sys,'Created');
      | if(isempty(first))
      |     first = datestr(now,'yyyy');
      | else
      |     first = first(end-3:end);  %year is last four digits
      | end
      | 
      | last = get_param(sys,'LastModifiedDate');
      | if isempty(last)
      |     last = datestr(now,'yyyy');
      | else
      |     last = last(end-3:end);
      | end
      | 
      | if strcmp(first,last)
      |     fprintf('%s -- Copyright %s Nexteer',NxtrConf,first)
      | else
      |     fprintf('%s -- %s%s- %s Nexteer',NxtrConf,char(169),first,last)
      | end
  Merge4 : Merge  Inputs=3
  Relational Operator2 : RelationalOperator  RequirementInfo="{'linktype_rmi_doors' '0000c6e0 (/GM T1XX/SubSystem Specifications/Customer Functions/CF012 12V Start Stop)' '#190' 'true' 'REQ:  190' '' } %GIDa_ed42b956_acf8_48ad_9bc4_447af0128ae6"  Operator===  OutDataTypeStr=boolean
  Relational Operator4 : RelationalOperator  RequirementInfo="{'linktype_rmi_doors' '0000c6e0 (/GM T1XX/SubSystem Specifications/Customer Functions/CF012 12V Start Stop)' '#191' 'true' 'REQ:  191' '' } %GIDa_11925cc0_82ac_48e6_b518_87c4cde2e70f"  Operator===  OutDataTypeStr=boolean
  StopMod_IF : If  RequirementInfo="{'linktype_rmi_doors' '0000c6e0 (/GM T1XX/SubSystem Specifications/Customer Functions/CF012 12V Start Stop)' '#190' 'true' 'REQ:  190' '' ; 'linktype_rmi_doors' '0000c6e0 (/GM T1XX/SubSystem Specifications/Customer Functions/CF012 12V Start Stop)' '#191' 'true' 'REQ:  191' '' ; 'linktype_rmi_doors' '0000c6e0 (/GM T1XX/SubSystem Specifications/Customer Functions/CF012 12V Start Stop)' '#196' 'true' 'REQ:  196' '' } %GIDa_bb67e0a1_8e4e_455e_a4e9_af7536b7ef1b"  NumInputs=2  IfExpression=u1  ElseIfExpressions=u2
  THEN1 : Subsystem  RequirementInfo="{'linktype_rmi_doors' '0000c6e0 (/GM T1XX/SubSystem Specifications/Customer Functions/CF012 12V Start Stop)' '#191' 'true' 'REQ:  191' '' } %GIDa_65b322e5_28d3_4828_b631_5c66e629d928"  TreatAsAtomicUnit=on  mask(pass thru, version Nov 30, 2012){nIn=1}
      mask prompts: nIn "Number of input signals"
      mask help:
      | This block passes its input straight through without modification.
      |
      | Enter the number of signals to pass through (integer 1 to 5).
      mask Callback nIn:
      | thisBlock = gcb;
      | a = get_param(thisBlock,'MaskValues');
      | b = cell2mat(a);
      | c = str2num(b);
      | 
      | if c<1 c=1; end
      | if c>5 c=5; end
      | 
      | for idx=1:c
      |     sIdx = num2str(idx);
      |     oldblock = [thisBlock '/In' sIdx];
      |     if strcmp(get_param(oldblock,'BlockType'),'Ground')
      |          newblock = 'built-in/Inport';
      |         pos = get_param(oldblock,'Position');
      |         orient = get_param(oldblock,'Orientation');
      |         delete_block(oldblock);
      |         add_block(newblock,oldblock,'Position',pos, 'Orientation',orient);
      |     end
      | 
      |     oldblock = [thisBlock '/Out' sIdx];
      |     if strcmp(get_param(oldblock,'BlockType'),'Terminator')
      |         newblock = 'built-in/Outport';
      |         pos = get_param(oldblock,'Position');
      |         orient = get_param(oldblock,'Orientation');
      |         delete_block(oldblock);
      |         add_block(newblock,oldblock,'Position',pos, 'Orientation',orient);
      |     end
      | end
      | 
      | for idx=c+1:5
      |     sIdx = num2str(idx);
      |     oldblock = [thisBlock '/In' sIdx];
      |     if strcmp(get_param(oldblock,'BlockType'),'Inport')
      |         newblock = 'built-in/Ground';
      |         pos = get_param(oldblock,'Position');
      |         orient = get_param(oldblock,'Orientation');
      |         delete_block(oldblock);
      |         add_block(newblock,oldblock,'Position',pos, 'Orientation',orient);
      |     end
      | 
      |     oldblock = [thisBlock '/Out' sIdx];
      |     if strcmp(get_param(oldblock,'BlockType'),'Outport')
      |         newblock = 'built-in/Terminator';
      |         pos = get_param(oldblock,'Position');
      |         orient = get_param(oldblock,'Orientation');
      |         delete_block(oldblock);
      |         add_block(newblock,oldblock,'Position',pos, 'Orientation',orient);
      |     end
      | end
      | 
      | 
      | 
      | clear thisBlock oldblock newblock orient pos a b c idx sIdx ;
      mask Display: fprintf('pass\nthru')
  THEN4 : Subsystem  RequirementInfo="{'linktype_rmi_doors' '0000c6e0 (/GM T1XX/SubSystem Specifications/Customer Functions/CF012 12V Start Stop)' '#190' 'true' 'REQ:  190' '' } %GIDa_a655192f_5a53_4590_9352_ed586a5ad0c6"  TreatAsAtomicUnit=on  mask(pass thru, version Nov 30, 2012){nIn=1}
      mask prompts: nIn "Number of input signals"
      mask help:
      | This block passes its input straight through without modification.
      |
      | Enter the number of signals to pass through (integer 1 to 5).
      mask Callback nIn:
      | thisBlock = gcb;
      | a = get_param(thisBlock,'MaskValues');
      | b = cell2mat(a);
      | c = str2num(b);
      | 
      | if c<1 c=1; end
      | if c>5 c=5; end
      | 
      | for idx=1:c
      |     sIdx = num2str(idx);
      |     oldblock = [thisBlock '/In' sIdx];
      |     if strcmp(get_param(oldblock,'BlockType'),'Ground')
      |          newblock = 'built-in/Inport';
      |         pos = get_param(oldblock,'Position');
      |         orient = get_param(oldblock,'Orientation');
      |         delete_block(oldblock);
      |         add_block(newblock,oldblock,'Position',pos, 'Orientation',orient);
      |     end
      | 
      |     oldblock = [thisBlock '/Out' sIdx];
      |     if strcmp(get_param(oldblock,'BlockType'),'Terminator')
      |         newblock = 'built-in/Outport';
      |         pos = get_param(oldblock,'Position');
      |         orient = get_param(oldblock,'Orientation');
      |         delete_block(oldblock);
      |         add_block(newblock,oldblock,'Position',pos, 'Orientation',orient);
      |     end
      | end
      | 
      | for idx=c+1:5
      |     sIdx = num2str(idx);
      |     oldblock = [thisBlock '/In' sIdx];
      |     if strcmp(get_param(oldblock,'BlockType'),'Inport')
      |         newblock = 'built-in/Ground';
      |         pos = get_param(oldblock,'Position');
      |         orient = get_param(oldblock,'Orientation');
      |         delete_block(oldblock);
      |         add_block(newblock,oldblock,'Position',pos, 'Orientation',orient);
      |     end
      | 
      |     oldblock = [thisBlock '/Out' sIdx];
      |     if strcmp(get_param(oldblock,'BlockType'),'Outport')
      |         newblock = 'built-in/Terminator';
      |         pos = get_param(oldblock,'Position');
      |         orient = get_param(oldblock,'Orientation');
      |         delete_block(oldblock);
      |         add_block(newblock,oldblock,'Position',pos, 'Orientation',orient);
      |     end
      | end
      | 
      | 
      | 
      | clear thisBlock oldblock newblock orient pos a b c idx sIdx ;
      mask Display: fprintf('pass\nthru')
  THEN5 : Subsystem  RequirementInfo="{'linktype_rmi_doors' '0000c6e0 (/GM T1XX/SubSystem Specifications/Customer Functions/CF012 12V Start Stop)' '#196' 'true' 'REQ:  196' '' } %GIDa_5f14c36c_f47b_462f_b360_b82b997058cc"  TreatAsAtomicUnit=on  mask(pass thru, version Nov 30, 2012){nIn=1}
      mask prompts: nIn "Number of input signals"
      mask help:
      | This block passes its input straight through without modification.
      |
      | Enter the number of signals to pass through (integer 1 to 5).
      mask Callback nIn:
      | thisBlock = gcb;
      | a = get_param(thisBlock,'MaskValues');
      | b = cell2mat(a);
      | c = str2num(b);
      | 
      | if c<1 c=1; end
      | if c>5 c=5; end
      | 
      | for idx=1:c
      |     sIdx = num2str(idx);
      |     oldblock = [thisBlock '/In' sIdx];
      |     if strcmp(get_param(oldblock,'BlockType'),'Ground')
      |          newblock = 'built-in/Inport';
      |         pos = get_param(oldblock,'Position');
      |         orient = get_param(oldblock,'Orientation');
      |         delete_block(oldblock);
      |         add_block(newblock,oldblock,'Position',pos, 'Orientation',orient);
      |     end
      | 
      |     oldblock = [thisBlock '/Out' sIdx];
      |     if strcmp(get_param(oldblock,'BlockType'),'Terminator')
      |         newblock = 'built-in/Outport';
      |         pos = get_param(oldblock,'Position');
      |         orient = get_param(oldblock,'Orientation');
      |         delete_block(oldblock);
      |         add_block(newblock,oldblock,'Position',pos, 'Orientation',orient);
      |     end
      | end
      | 
      | for idx=c+1:5
      |     sIdx = num2str(idx);
      |     oldblock = [thisBlock '/In' sIdx];
      |     if strcmp(get_param(oldblock,'BlockType'),'Inport')
      |         newblock = 'built-in/Ground';
      |         pos = get_param(oldblock,'Position');
      |         orient = get_param(oldblock,'Orientation');
      |         delete_block(oldblock);
      |         add_block(newblock,oldblock,'Position',pos, 'Orientation',orient);
      |     end
      | 
      |     oldblock = [thisBlock '/Out' sIdx];
      |     if strcmp(get_param(oldblock,'BlockType'),'Outport')
      |         newblock = 'built-in/Terminator';
      |         pos = get_param(oldblock,'Position');
      |         orient = get_param(oldblock,'Orientation');
      |         delete_block(oldblock);
      |         add_block(newblock,oldblock,'Position',pos, 'Orientation',orient);
      |     end
      | end
      | 
      | 
      | 
      | clear thisBlock oldblock newblock orient pos a b c idx sIdx ;
      mask Display: fprintf('pass\nthru')
  StrtStopRateLim : Outport
  wires:
  Constant8/1 -> THEN4/1(In1)
  Constant5/1 -> THEN1/1(In1)
  Merge4/1 -> StrtStopRateLim/1
  StopMod_IF/2 -> THEN4/Action
  THEN1/1(Out1) -> Merge4/1
  THEN4/1(Out1) -> Merge4/2
  StopMod_IF/1 -> THEN1/Action
  THEN5/1(Out1) -> Merge4/3
  StopMod_IF/3 -> THEN5/Action
  Constant7/1 -> THEN5/1(In1)
  StrtStopSt/1 -> Relational Operator2/1, Relational Operator4/1
  Constant3/1 -> Relational Operator2/2
  Constant1/1 -> Relational Operator4/2
  Relational Operator4/1 -> StopMod_IF/1
  Relational Operator2/1 -> StopMod_IF/2

== system CF012A_GmStrtStop/GmStrtStop/GmStrtStopPer1/Inter1ToStopModFlg/CopyRight2 ==
